simulink model "SiEngineController"  (R2021a)
settings: Solver=ode4  StartTime=0.0  StopTime=inf  FixedStep=.01  RelTol=1e-3  EnableMultiTasking=on
model workspace (MAT data in the model file):
  CatLightOffTime = 0
  Cps = 2
  CrankSpeed = 150
  EngRevLim = 7000
  EngStopStartEnable = 1
  EngStopTime : Simulink.Parameter (value not decoded)
  NCyl = 4
  N_idle = 750
  Pstd = 101325
  Rair = 287
  Sinj = 6.45161290323
  Ts : Simulink.Parameter (value not decoded)
  Tstd = 293.15
  Vd = 0.0015
  afr_stoich = 14.6
  calEngVar : object (value not decoded)
  f_cp_ld_bpt = [0 0.2 0.275 0.35 0.425 0.5 0.575 0.65 0.725 0.8 0.875 0.95 ... (16 elements, 1x16)]
  f_cp_n_bpt = [750 1053.57142857 1357.14285714 1660.71428571 1964.28571429 2267.85714286 2571.42857143 2875 3178.57142857 3482.14285714 3785.71428571 4089.28571429 ... (15 elements, 1x15)]
  f_del_sa_bpt = [0 0.75 1.5 2.25 3 3.75 4.5 5.25 6 6.75 7.5 8.25 ... (65 elements, 1x65)]
  f_ecp = [0 0 7.19012817097 15.3709456879 19.1470470057 19.0854874367 13.5819971805 0 0 0 0 0 ... (240 elements, 16x15)]
  f_egr_areapct_cmd = [0 3.448 6.897 10.34 13.79 17.24 20.69 24.14 27.59 31.03 34.48 37.93 ... (600 elements, 30x20)]
  f_egr_areapct_nrmlzdflow_bpt = [0 0.03448 0.06897 0.1034 0.1379 0.1724 0.2069 0.2414 0.2759 0.3103 0.3448 0.3793 ... (30 elements, 1x30)]
  f_egr_areapct_pr_bpt = [0.5 0.5263 0.5526 0.5789 0.6053 0.6316 0.6579 0.6842 0.7105 0.7368 0.7632 0.7895 ... (20 elements, 20x1)]
  f_egr_max_stdflow = [74.87 74.87 74.74 74.39 73.81 72.98 71.91 70.58 68.97 67.06 64.84 62.25 ... (20 elements, 1x20)]
  f_egr_stdflow = [0 3.743 7.487 11.23 14.97 18.72 22.46 26.2 29.95 33.69 37.43 41.18 ... (420 elements, 21x20)]
  f_egr_stdflow_egrap_bpt = [0 5 10 15 20 25 30 35 40 45 50 55 ... (21 elements, 21x1)]
  f_egr_stdflow_pr_bpt = [0.5 0.5263 0.5526 0.5789 0.6053 0.6316 0.6579 0.6842 0.7105 0.7368 0.7632 0.7895 ... (20 elements, 20x1)]
  f_egrpct_cmd = [0 0 0 0 0 0 0 0 0 0 0 0 ... (240 elements, 16x15)]
  f_egrpct_ld_bpt = [0 0.2 0.275 0.35 0.425 0.5 0.575 0.65 0.725 0.8 0.875 0.95 ... (16 elements, 1x16)]
  f_egrpct_n_bpt = [750 1054 1357 1661 1964 2268 2571 2875 3179 3482 3786 4089 ... (15 elements, 1x15)]
  f_fric_temp_bpt = [274 276 278 280 282 284 286 288 290 292 294 296 ... (54 elements, 1x54)]
  f_fric_temp_mod = [3.96 3.22 2.56 2.26 2.11 2 1.9 1.83 1.76 1.7 1.65 1.6 ... (54 elements, 1x54)]
  f_icp = [0 0 1 1.09273642197 2.29409401139 3.54274371837 0.947749647567 0 0 0 0 0 ... (240 elements, 16x15)]
  f_intksys_stdflow_bpt = [0 29.67 59.34 89.01 117.8 144.1 155.7 166 175.2 183.3 190.7 197 ... (20 elements, 1x20)]
  f_intksys_stdflow_pr = [1 0.9789 0.9579 0.9368 0.9158 0.8947 0.8737 0.8526 0.8316 0.8105 0.7895 0.7684 ... (20 elements, 1x20)]
  f_lamcmd = [1 1 1 1 1 1 1 1 1 1 1 1 ... (240 elements, 16x15)]
  f_lamcmd_ld_bpt = [0 0.2 0.275 0.35 0.425 0.5 0.575 0.65 0.725 0.8 0.875 0.95 ... (16 elements, 1x16)]
  f_lamcmd_n_bpt = [750 1053.57142857 1357.14285714 1660.71428571 1964.28571429 2267.85714286 2571.42857143 2875 3178.57142857 3482.14285714 3785.71428571 4089.28571429 ... (15 elements, 1x15)]
  f_lcmd = [0 0.191691264188 0.286571334902 0.358602176134 0.434951283804 0.517809198874 0.591334436539 0.614814588717 0.614814588717 0.614814588717 0.614814588717 0.614814588717 ... (315 elements, 21x15)]
  f_lcmd_n_bpt = [750 1053.57142857 1357.14285714 1660.71428571 1964.28571429 2267.85714286 2571.42857143 2875 3178.57142857 3482.14285714 3785.71428571 4089.28571429 ... (15 elements, 1x15)]
  f_lcmd_tq_bpt = [0 15 26.3157894737 37.6315789474 48.9473684211 60.2631578947 71.5789473684 82.8947368421 94.2105263158 105.526315789 116.842105263 128.157894737 ... (21 elements, 1x21)]
  f_m_lam = [0.94128 0.95565 0.97001 0.98437 0.99008 1.0004 0.97527 0.9549 0.92612 0.89735 0]
  f_m_lam_bpt = [0.65 0.7 0.75 0.8 0.85 0.9 0.95 1 1.05 1.1 2]
  f_m_sa = [1.0019 0.9988 0.9953 0.99173 0.98811 0.98441 0.98065 0.97682 0.97293 0.96897 0.96493 0.96083 ... (65 elements, 1x65)]
  f_mdot_air_corr = [1.02156051768 1.00597426471 0.989411677851 1.0033499089 0.984591437857 0.988509040623 1.0326198627 1.02765527362 1.0134784519 0.998280021213 0.981755128787 0.967218261288 ... (400 elements, 20x20)]
  f_mdot_air_corr_ld_bpt = [0.223381333333 0.285105122807 0.346828912281 0.408552701754 0.470276491228 0.532000280702 0.593724070175 0.655447859649 0.717171649123 0.778895438596 0.84061922807 0.902343017544 ... (20 elements, 1x20)]
  f_mdot_air_n_bpt = [750 973.6842 1197.3684 1421.0526 1644.7368 1868.4211 2092.1053 2315.7895 2539.4737 2763.1579 2986.8421 3210.5263 ... (20 elements, 1x20)]
  f_mdot_intk = [0 0 0 0 0 0 0 0 0 0 0 0 ... (400 elements, 20x20)]
  f_mdot_intk_ecp_bpt = [0 2.6316 5.2632 7.8947 10.5263 13.1579 15.7895 18.4211 21.0526 23.6842 26.3158 28.9474 ... (20 elements, 1x20)]
  f_mdot_trpd_bpt = [0 5.7895 11.5789 17.3684 23.1579 28.9474 34.7368 40.5263 46.3158 52.1053 57.8947 63.6842 ... (20 elements, 1x20)]
  f_nv = [0.64175366561 0.641419295169 0.640125365558 0.638690556197 0.644169906538 0.669178791311 0.731659452876 0.750078238889 0.750078238889 0.750078238889 0.750078238889 0.750078238889 ... (225 elements, 15x15)]
  f_nv_n_bpt = [750 1053.57142857 1357.14285714 1660.71428571 1964.28571429 2267.85714286 2571.42857143 2875 3178.57142857 3482.14285714 3785.71428571 4089.28571429 ... (15 elements, 1x15)]
  f_nv_prs_bpt = [31 40.6428571429 50.2857142857 59.9285714286 69.5714285714 79.2142857143 88.8571428571 98.5 108.142857143 117.785714286 127.428571429 137.071428571 ... (15 elements, 1x15)]
  f_sa = [9.05 9.05 16.4373253582 15.3405265461 13.6074880273 9.83352189562 3.89388784387 0 0 0 0 0 ... (240 elements, 16x15)]
  f_sa_ld_bpt = [0 0.2 0.275 0.35 0.425 0.5 0.575 0.65 0.725 0.8 0.875 0.95 ... (16 elements, 1x16)]
  f_sa_n_bpt = [750 1053.57142857 1357.14285714 1660.71428571 1964.28571429 2267.85714286 2571.42857143 2875 3178.57142857 3482.14285714 3785.71428571 4089.28571429 ... (15 elements, 1x15)]
  f_sa_opt = [9.05 9.05 16.4373253582 15.3405265461 13.6074880273 9.83352189562 3.89388784387 2.22044604925e-16 2.22044604925e-16 2.22044604925e-16 2.22044604925e-16 2.22044604925e-16 ... (256 elements, 16x16)]
  f_startup_ect_bpt = [-40 0 20 50]
  f_startup_lambda_delta = [0.5 0.3 0.2 0]
  f_startup_lambda_delta_timecnst = [90 40 12 0]
  f_t_exh = [739.936218766 750.584766028 772.770773797 791.235245621 803.106549716 885.862998064 920.498479307 920.498479307 920.498479307 920.498479307 920.498479307 920.498479307 ... (225 elements, 15x15)]
  f_t_exh_l_bpt = [0.2 0.275 0.35 0.425 0.5 0.575 0.65 0.725 0.8 0.875 0.95 1.025 ... (15 elements, 1x15)]
  f_t_exh_n_bpt = [750 1053.57142857 1357.14285714 1660.71428571 1964.28571429 2267.85714286 2571.42857143 2875 3178.57142857 3482.14285714 3785.71428571 4089.28571429 ... (15 elements, 1x15)]
  f_tap = [0 0.526932471044 0.76956291542 0.98216380025 1.2334307097 1.55068264267 2.00046965195 2.58135641722 2.62499999998 2.62499999998 2.62499999998 2.62499999998 ... (315 elements, 21x15)]
  f_tap_ld_bpt = [0 0.2 0.268421052632 0.336842105263 0.405263157895 0.473684210526 0.542105263158 0.610526315789 0.678947368421 0.747368421053 0.815789473684 0.884210526316 ... (21 elements, 1x21)]
  f_tap_n_bpt = [750 1053.57142857 1357.14285714 1660.71428571 1964.28571429 2267.85714286 2571.42857143 2875 3178.57142857 3482.14285714 3785.71428571 4089.28571429 ... (15 elements, 1x15)]
  f_tm_corr = [0.839360054391 0.833393271885 0.82629554201 0.818442814437 0.811524387436 0.809164184856 0.814606352881 0.826887956871 0.842304598924 0.856886829014 0.869487025783 0.880530414174 ... (400 elements, 20x20)]
  f_tm_corr_n_bpt = [750 973.6842 1197.3684 1421.0526 1644.7368 1868.4211 2092.1053 2315.7895 2539.4737 2763.1579 2986.8421 3210.5263 ... (20 elements, 1x20)]
  f_tm_corr_nd_bpt = [0.3 0.38947 0.47895 0.56842 0.65789 0.74737 0.83684 0.92632 1.0158 1.1053 1.1947 1.2842 ... (20 elements, 1x20)]
  f_tpp = [0 100]
  f_tpp_tap_bpt = [0 100]
  f_tq_fric = [0 0 0 0 0 0 0 0 0 0 0 0 ... (256 elements, 16x16)]
  f_tq_inr = [25.8508 25.8508 31 37 43 50 50 50 50 50 50 50 ... (256 elements, 16x16)]
  f_tq_inr_l_bpt = [0.1 0.2 0.28571 0.37143 0.45714 0.54286 0.62857 0.71429 0.8 0.88571 0.97143 1.0571 ... (16 elements, 1x16)]
  f_tq_inr_n_bpt = [0 750 1053.5714 1357.1429 1660.7143 1964.2857 2267.8571 2571.4286 2875 3178.5714 3482.1429 3785.7143 ... (16 elements, 1x16)]
  f_tq_nl = [0 15.0012133443 26.4298333923 37.8556656512 49.2846782956 60.7113978793 72.3451969202 77.459652163 78.5324534074 78.5324534074 78.5324534074 78.5324534074 ... (256 elements, 16x16)]
  f_tq_nl_l_bpt = [0 0.2 0.275 0.35 0.425 0.5 0.575 0.65 0.725 0.8 0.875 0.95 ... (16 elements, 1x16)]
  f_tq_nl_n_bpt = [0 750 1053.57142857 1357.14285714 1660.71428571 1964.28571429 2267.85714286 2571.42857143 2875 3178.57142857 3482.14285714 3785.71428571 ... (16 elements, 1x16)]
  f_tq_pump = [0 0 0 0 0 0 0 0 0 0 0 0 ... (256 elements, 16x16)]
  f_vivc = [0.37716 0.38164 0.38611 0.39033 0.39428 0.39795 0.40132 0.40441 0.40719 0.40967 0.41184 0.41372 ... (20 elements, 1x20)]
  f_vivc_icp_bpt = [0 2.6316 5.2632 7.8947 10.5263 13.1579 15.7895 18.4211 21.0526 23.6842 26.3158 28.9474 ... (20 elements, 1x20)]
  f_wap = [100 100 100 100 100 100 100 100 100 100 100 100 ... (315 elements, 21x15)]
  f_wap_ld_bpt = [0 0.2 0.268421052632 0.336842105263 0.405263157895 0.473684210526 0.542105263158 0.610526315789 0.678947368421 0.747368421053 0.815789473684 0.884210526316 ... (21 elements, 1x21)]
  f_wap_n_bpt = [750 1053.57142857 1357.14285714 1660.71428571 1964.28571429 2267.85714286 2571.42857143 2875 3178.57142857 3482.14285714 3785.71428571 4089.28571429 ... (15 elements, 1x15)]
  tau_egr = 0.2
symbols that are objects in the model workspace (value not decoded): EngStopTime, Ts
libraries: simulink x3, autolibengctrlr x1
(part 2 of 2)

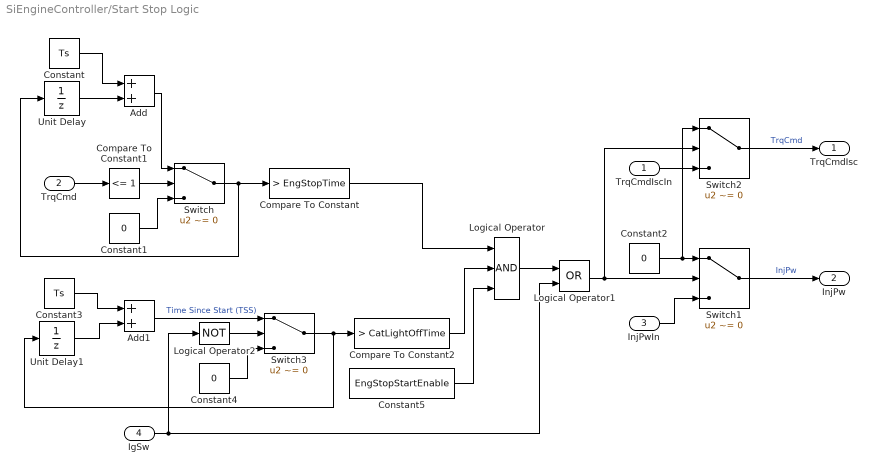
== system SiEngineController/Start Stop Logic ==
  TrqCmdIscIn : Inport
  TrqCmd : Inport  Port=2
  InjPwIn : Inport  Port=3
  IgSw : Inport  Port=4
  Add : Sum
  Add1 : Sum
  Compare To Constant : simulink/Logic and Bit Operations/Compare To Constant  relop=>  const=EngStopTime  OutDataTypeStr=boolean
  Compare To Constant1 : simulink/Logic and Bit Operations/Compare To Constant  relop=<=  const=1  OutDataTypeStr=boolean
  Compare To Constant2 : simulink/Logic and Bit Operations/Compare To Constant  relop=>  const=CatLightOffTime  OutDataTypeStr=boolean
  Constant : Constant  Value=Ts
  Constant1 : Constant  Value=0
  Constant2 : Constant  Value=0
  Constant3 : Constant  Value=Ts
  Constant4 : Constant  Value=0
  Constant5 : Constant  Value=EngStopStartEnable
  Logical Operator : Logic  Inputs=3  AllPortsSameDT=off  OutDataTypeStr=boolean
  Logical Operator1 : Logic  Operator=OR  AllPortsSameDT=off  OutDataTypeStr=boolean
  Logical Operator2 : Logic  Operator=NOT  AllPortsSameDT=off  OutDataTypeStr=boolean
  Switch{,1..3} (4 alike) : Switch  Criteria=u2 ~= 0
  Unit Delay : UnitDelay  InitialCondition=EngStopTime+1  SampleTime=-1  HasFrameUpgradeWarning=on
  Unit Delay1 : UnitDelay  InitialCondition=CatLightOffTime+1  SampleTime=-1  HasFrameUpgradeWarning=on
  TrqCmdIsc : Outport  VectorParamsAs1DForOutWhenUnconnected=off
  InjPw : Outport  Port=2  VectorParamsAs1DForOutWhenUnconnected=off
  wires:
  Unit Delay/1 -> Add/2
  Add/1 -> Switch/1
  Constant/1 -> Add/1
  Logical Operator1/1 -> Switch1/2, Switch2/2
  Compare To Constant1/1 -> Switch/2
  TrqCmd/1 -> Compare To Constant1/1
  Switch/1 -> Compare To Constant/1, Unit Delay/1
  Constant1/1 -> Switch/3
  Constant2/1 -> Switch2/1, Switch1/1
  InjPwIn/1 -> Switch1/3
  Switch1/1 -> InjPw/1  "InjPw"
  TrqCmdIscIn/1 -> Switch2/3
  Switch2/1 -> TrqCmdIsc/1  "TrqCmd"
  Switch3/1 -> Unit Delay1/1, Compare To Constant2/1
  Add1/1 -> Switch3/1  "Time Since Start (TSS)"
  Constant4/1 -> Switch3/3
  Logical Operator2/1 -> Switch3/2
  Constant5/1 -> Logical Operator/3
  Unit Delay1/1 -> Add1/2
  Compare To Constant2/1 -> Logical Operator/2
  Constant3/1 -> Add1/1
  IgSw/1 -> Logical Operator2/1, Logical Operator1/2
  Compare To Constant/1 -> Logical Operator/1
  Logical Operator/1 -> Logical Operator1/1
